simulink model "Extended_Estimator"  (R2024b)
settings: Solver=VariableStepAuto  StartTime=0.0  StopTime=10.0  MaxStep=1e-4  RelTol=1e-3
values from neighbouring files (symbols this model uses):
  A = [0  1 ... (first row only)    [Ex1.m]    (also in Ex2.m; Ex3.m = [0 1; Extended_Estimator.m = [0 1)
  Ao = phi-L*H    [Ex2.m]    (also in Ex3.m; Extended_Estimator.m = Ae-L*Ce)
  B = [0 ... (first row only)    [Ex1.m]    (also in Ex2.m; Ex3.m; Extended_Estimator.m)
  Bo = [gamma L]    [Ex2.m]    (also in Ex3.m; Extended_Estimator.m = [Be L])
  C = [1 0]    [Ex1.m]    (also in Ex2.m = [90 0]; Ex3.m; Extended_Estimator.m)
  Co = eye(2)    [Ex2.m]    (also in Ex3.m; Extended_Estimator.m = eye(5))
  Do = zeros(2,2)    [Ex2.m]    (also in Ex3.m; Extended_Estimator.m = zeros(5,2))
  k = acker(phi, gamma,eigs_d)    [Ex2.m]    (also in Ex3.m = dlqr(phi_e,gamma_e,Q,R); Ex4.m = acker(A_z,B_z,eigs); Extended_Estimator.m = acker(A,B,pol_c))
  w = 6    [Ex4.m]    (also in Extended_Estimator.m)
settings Model: Creator=bmm1  LastModifiedBy=bmm1

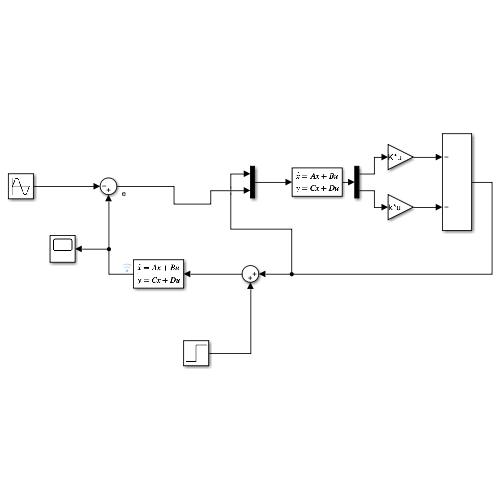
[thumbnail: Simulink's stored preview of the top-level diagram]
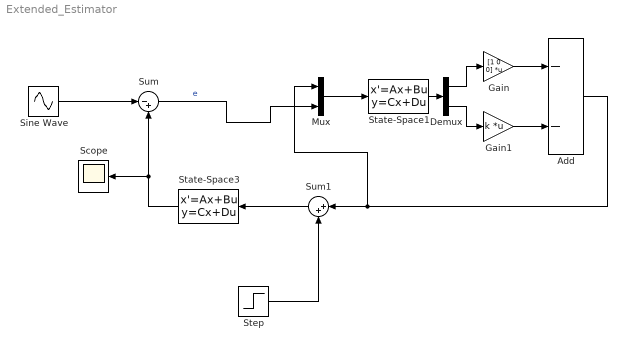
== system Extended_Estimator ==
  Add : Sum  Inputs=--
  Demux : Demux  Outputs=2
  Gain : Gain  Gain=[1 0 0]  Multiplication=Matrix(K*u)
  Gain1 : Gain  Gain=k  Multiplication=Matrix(K*u)
  Mux : Mux  Inputs=2
  Scope : Scope
  Sine Wave : Sin  Frequency=w  SampleTime=0
  State-Space1 : StateSpace  A=Ao  B=Bo  C=Co  D=Do  InitialCondition=0
  State-Space3 : StateSpace  A=A  B=B  C=C  D=0  InitialCondition=0
  Step : Step  SampleTime=0
  Sum : Sum  Inputs=|-+
  Sum1 : Sum  Inputs=|++
  wires:
  Sine Wave/1 -> Sum/1
  State-Space3/1 -> Scope/1, Sum/2
  Sum1/1 -> State-Space3/1
  Add/1 -> Mux/1, Sum1/1
  Mux/1 -> State-Space1/1
  Gain/1 -> Add/1
  Gain1/1 -> Add/2
  Step/1 -> Sum1/2
  State-Space1/1 -> Demux/1
  Demux/1 -> Gain/1
  Demux/2 -> Gain1/1
  Sum/1 -> Mux/2  "e"
